simulink model "GFLIB_ControllerPIp_BAM"  (Simulink 9.3)
settings: Solver=VariableStepAuto  StartTime=0.0  StopTime=10.0  RelTol=1e-3
settings Model: Creator=nxa18952  LastModifiedBy=nxa18952
settings DataIOCC: SaveFormat=Dataset  SignalLoggingSaveFormat=Dataset  ReturnWorkspaceOutputs=on
settings OptimizationCC: LifeSpan=auto
settings DebuggingCC: UnderspecifiedInitializationDetection=Simplified  MergeDetectMultiDrivingBlocksExec=error  FcnCallInpInsideContextMsg=error  SFUnexpectedBacktrackingDiag=error  SFNoUnconditionalDefaultTransitionDiag=error  SFExecutionAtInitializationDiag=warning  ArithmeticOperatorsInVariantConditions=error
settings HardwareCC: ProdBitPerPointer=64  ProdBitPerSizeT=64  ProdBitPerPtrDiffT=64  ProdLargestAtomicFloat=Float  ProdIntDivRoundTo=Zero  ProdEndianess=LittleEndian  ProdWordSize=64  ProdHWDeviceType=Intel->x86-64 (Windows64)
settings ModelReferenceCC: PropagateSignalLabelsOutOfModel=on
settings SFSimCC: SimUseLocalCustomCode=on
settings RTWCC: RTWUseLocalCustomCode=on
settings CodeAppCC: StateflowObjectComments=off
settings GRTTargetCC: TargetLangStandard=C99 (ISO)  CombineOutputUpdateFcns=on  GRTInterface=off
settings ConfigComp: CovMetricSettings=dwe  CovHtmlReporting=off  CovSaveCumulativeToWorkspaceVar=off  CovSaveSingleToWorkspaceVar=off  CovExternalEMLEnable=on

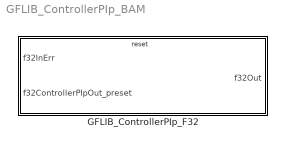
== system GFLIB_ControllerPIp_BAM ==
  GFLIB_ControllerPIp_F32 : Subsystem  TreatAsAtomicUnit=on  mask(GFLIB_ControllerPIp_F32){showStates=Hide (faster execution), resetStatesEnable=Pre-set according to the first set of inputs after reset, f32PropGain=0, f32IntegGain=0, s16PropGainShift=0, s16IntegGainShift=0}
      mask prompts: showStates "Show internal states"; resetStatesEnable "Internal state after reset"; f32PropGain "f32PropGain (Proportional gain)"; f32IntegGain "f32IntegGain (Integral gain)"; s16PropGainShift "s16PropGainShift (Proportional gain shift)"; s16IntegGainShift "s16IntegGainShift (Integral gain shift)"
      mask help: Parallel form PI controller without anti-windup in 32-bit fixed-point fractional implementation. This block supports re-initialization of the internal state during simulation. If the block is reset, the controller's output will be aligned with the input f32ControllerPIpOut_preset. Refer to the AMMCLIB User's Guide for further details.
      mask init:
      | if ~evalin('base','exist(''tS8'',''var'')')
      |   if (2 ~= exist('SWLIBS_Typedefs.mat','file'))
      |       error('File SWLIBS_Typedefs.mat is not on the Matlab path. Please add the AMMCLIB "bam" folder in the Matlab Search Path.');
      |   else
      |       evalin('base', 'load(''SWLIBS_Typedefs.mat'')');
      |   end
      | end
      | if showStates == 1
      |     % hidden state variables
      |     if strcmp(get_param([gcb '/f32PropGain'], 'BlockType'), 'Inport')
      |         posblk = get_param(gcb, 'Position');
      | 
      |         pos = get_param(    [gcb, '/f32PropGain'], 'Position');
      |         orient = get_param( [gcb, '/f32PropGain'], 'Orientation');
      |         delete_block(       [gcb, '/f32PropGain']);
      |         add_block('built-in/Ground', [gcb, '/f32PropGain'], 'Position', pos, 'Orientation', orient);
      | 
      |         pos = get_param(    [gcb, '/f32IntegGain'], 'Position');
      |         orient = get_param( [gcb, '/f32IntegGain'], 'Orientation');
      |         delete_block(       [gcb, '/f32IntegGain']);
      |         add_block('built-in/Ground', [gcb, '/f32IntegGain'], 'Position', pos, 'Orientation', orient);
      | 
      |         pos = get_param(    [gcb, '/s16PropGainShift'], 'Position');
      |         orient = get_param( [gcb, '/s16PropGainShift'], 'Orientation');
      |         delete_block(       [gcb, '/s16PropGainShift']);
      |         add_block('built-in/Ground', [gcb, '/s16PropGainShift'], 'Position', pos, 'Orientation', orient);
      | 
      |         pos = get_param(    [gcb, '/s16IntegGainShift'], 'Position');
      |         orient = get_param( [gcb, '/s16IntegGainShift'], 'Orientation');
      |         delete_block(       [gcb, '/s16IntegGainShift']);
      |         add_block('built-in/Ground', [gcb, '/s16IntegGainShift'], 'Position', pos, 'Orientation', orient);
      | 
      |         pos = get_param(    [gcb, '/f32IntegPartK_1'], 'Position');
      |         orient = get_param( [gcb, '/f32IntegPartK_1'], 'Orientation');
      |         delete_block(       [gcb, '/f32IntegPartK_1']);
      |         add_block('built-in/Ground', [gcb, '/f32IntegPartK_1'], 'Position', pos, 'Orientation', orient);
      | 
      |         pos = get_param(    [gcb, '/f32InK_1'], 'Position');
      |         orient = get_param( [gcb, '/f32InK_1'], 'Orientation');
      |         delete_block(       [gcb, '/f32InK_1']);
      |         add_block('built-in/Ground', [gcb, '/f32InK_1'], 'Position', pos, 'Orientation', orient);
      | 
      | 
      |         pos = get_param(    [gcb '/f32IntegPartK_1_Out'], 'Position');
      |         orient = get_param( [gcb '/f32IntegPartK_1_Out'], 'Orientation');
      |         delete_block(       [gcb '/f32IntegPartK_1_Out']);
      |         add_block('built-in/Terminator', [gcb '/f32IntegPartK_1_Out'], 'Position', pos, 'Orientation', orient);
      | 
      |         pos = get_param(    [gcb '/f32InK_1_Out'], 'Position');
      |         orient = get_param( [gcb '/f32InK_1_Out'], 'Orientation');
      |         delete_block(       [gcb '/f32InK_1_Out']);
      |         add_block('built-in/Terminator', [gcb '/f32InK_1_Out'], 'Position', pos, 'Orientation', orient);
      | 
      | 
      |         set_param([gcb '/f32InErr'], 'Port', '1');
      |         set_param([gcb '/f32ControllerPIpOut_preset'], 'Port', '2');
      | 
      |         set_param([gcb '/f32Out'], 'Port', '1');
      | 
      |         set_param(gcb,'MaskEnables',{'on','on','on','on','on','on'});
      | 
      |         if (posblk(4) - posblk(2)) > 75
      |           height = 75;
      |           set_param(gcb,'Position',[posblk(1), posblk(2), posblk(3), posblk(2)+height])
      |         end
      |     end
      | else
      |     % shown state variables
      |     if strcmp(get_param([gcb '/f32PropGain'], 'BlockType'), 'Ground')
      |         posblk = get_param(gcb, 'Position');
      | 
      |         pos = get_param(    [gcb, '/f32PropGain'], 'Position');
      |         orient = get_param( [gcb, '/f32PropGain'], 'Orientation');
      |         delete_block(       [gcb, '/f32PropGain']);
      |         add_block('built-in/Inport', [gcb, '/f32PropGain'], 'Position', pos, 'Orientation', orient, 'OutDataTypeStr', 'int32');
      | 
      |         pos = get_param(    [gcb, '/f32IntegGain'], 'Position');
      |         orient = get_param( [gcb, '/f32IntegGain'], 'Orientation');
      |         delete_block(       [gcb, '/f32IntegGain']);
      |         add_block('built-in/Inport', [gcb, '/f32IntegGain'], 'Position', pos, 'Orientation', orient, 'OutDataTypeStr', 'int32');
      | 
      |         pos = get_param(    [gcb, '/s16PropGainShift'], 'Position');
      |         orient = get_param( [gcb, '/s16PropGainShift'], 'Orientation');
      |         delete_block(       [gcb, '/s16PropGainShift']);
      |         add_block('built-in/Inport', [gcb, '/s16PropGainShift'], 'Position', pos, 'Orientation', orient, 'OutDataTypeStr', 'int16');
      | 
      |         pos = get_param(    [gcb, '/s16IntegGainShift'], 'Position');
      |         orient = get_param( [gcb, '/s16IntegGainShift'], 'Orientation');
      |         delete_block(       [gcb, '/s16IntegGainShift']);
      |         add_block('built-in/Inport', [gcb, '/s16IntegGainShift'], 'Position', pos, 'Orientation', orient, 'OutDataTypeStr', 'int16');
      | 
      |         pos = get_param(    [gcb, '/f32IntegPartK_1'], 'Position');
      |         orient = get_param( [gcb, '/f32IntegPartK_1'], 'Orientation');
      |         delete_block(       [gcb, '/f32IntegPartK_1']);
      |         add_block('built-in/Inport', [gcb, '/f32IntegPartK_1'], 'Position', pos, 'Orientation', orient, 'OutDataTypeStr', 'int32');
      | 
      |         pos = get_param(    [gcb, '/f32InK_1'], 'Position');
      |         orient = get_param( [gcb, '/f32InK_1'], 'Orientation');
      |         delete_block(       [gcb, '/f32InK_1']);
      |         add_block('built-in/Inport', [gcb, '/f32InK_1'], 'Position', pos, 'Orientation', orient, 'OutDataTypeStr', 'int32');
      | 
      | 
      |         pos = get_param(    [gcb '/f32IntegPartK_1_Out'], 'Position');
      |         orient = get_param( [gcb '/f32IntegPartK_1_Out'], 'Orientation');
      |         delete_block(       [gcb '/f32IntegPartK_1_Out']);
      |         add_block('built-in/Outport', [gcb '/f32IntegPartK_1_Out'], 'Position', pos, 'Orientation', orient);
      | 
      |         pos = get_param(    [gcb '/f32InK_1_Out'], 'Position');
      |         orient = get_param( [gcb '/f32InK_1_Out'], 'Orientation');
      |         delete_block(       [gcb '/f32InK_1_Out']);
      |         add_block('built-in/Outport', [gcb '/f32InK_1_Out'], 'Position', pos, 'Orientation', orient);
      | 
      | 
      |         set_param([gcb '/f32InErr'], 'Port', '1');
      |         set_param([gcb '/f32ControllerPIpOut_preset'], 'Port', '2');
      |         set_param([gcb '/f32PropGain'], 'Port', '3');
      |         set_param([gcb '/f32IntegGain'], 'Port', '4');
      |         set_param([gcb '/s16PropGainShift'], 'Port', '5');
      |         set_param([gcb '/s16IntegGainShift'], 'Port', '6');
      |         set_param([gcb '/f32IntegPartK_1'], 'Port', '7');
      |         set_param([gcb '/f32InK_1'], 'Port', '8');
      | 
      |         set_param([gcb '/f32Out'], 'Port', '1');
      |         set_param([gcb '/f32IntegPartK_1_Out'], 'Port', '2');
      |         set_param([gcb '/f32InK_1_Out'], 'Port', '3');
      | 
      |         set_param(gcb,'MaskEnables',{'on','on','off','off','off','off'});
      | 
      |         if (posblk(4) - posblk(2)) < 225
      |           height = 225;
      |           set_param(gcb,'Position',[posblk(1), posblk(2), posblk(3), posblk(2)+height])
      |         end
      |     end
      | end
      settings: RTWSystemCode=Inline
      mask TypeOptions showStates: Hide (faster execution) | Show (allows debugging; connect feedback loops manually)
      mask Callback showStates:
      | maskStr = get_param(gcb,'showStates');
      | if strcmp(maskStr,'Hide (faster execution)'),
      |     set_param(gcb,'MaskEnables',{'on','on','on','on','on','on'});
      | else
      |     set_param(gcb,'MaskEnables',{'on','on','off','off','off','off'});
      | end
      mask TypeOptions resetStatesEnable: Pre-set according to the first set of inputs after reset | Clear to zero
      mask Display:
      | color('black');
      | pos = get_param(gcb, 'Position');
      | width = pos(3) - pos(1);
      | height = pos(4) - pos(2);
      | tX=width/2;
      | tY=height - 25;
      | color('black');
      | text(tX,tY, 'GFLIB_ControllerPIp_F32', 'horizontalAlignment', 'center');
      | if showStates == 2
      |   color('red');
      |   text(tX,tY - 20, ['debugging mode' char(13) char(10) '(limited performance)'], 'horizontalAlignment', 'center');
      | end

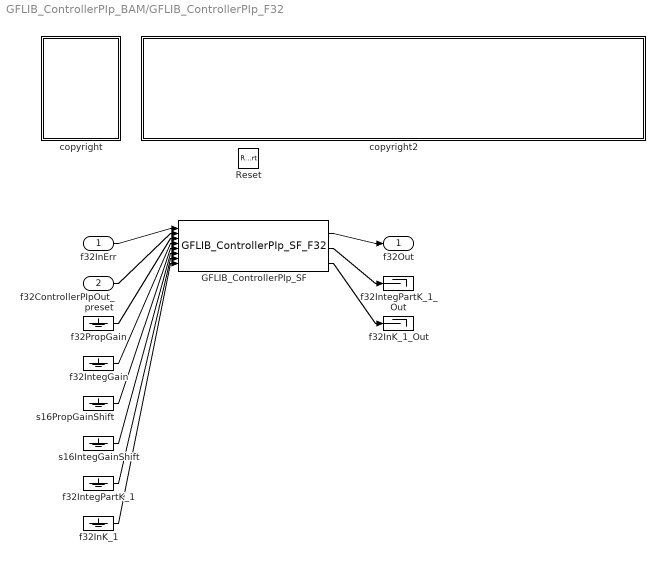
== system GFLIB_ControllerPIp_BAM/GFLIB_ControllerPIp_F32 ==
  f32InErr : Inport  OutDataTypeStr=int32
  f32ControllerPIpOut_preset : Inport  Port=2  OutDataTypeStr=int32
  Reset : ResetPort  DisableCoverage=on
  GFLIB_ControllerPIp_SF : S-Function  FunctionName=GFLIB_ControllerPIp_SF_F32  Parameters=showStates,resetStatesEnable,f32PropGain,f32IntegGain,s16PropGainShift,s16IntegGainShift  SFunctionDeploymentMode=off  EnableBusSupport=off
  copyright : Subsystem
      mask Display: text(10,90,'FILE:');text(10,75,'DESRIPTION:');text(10,60,'COPYRIGHT:');text(10,45,'VERSION:');text(10,30,'DATE:')
  copyright2 : Subsystem
      mask Display: text(10,90,'GFLIB_ControllerPIp_BAM_F32.mdl');text(10,75,'Parallel form of a standard PI controller without anti-windup.');text(10,60,'NXP 2020');text(10,45,'1.0');text(10,30,'28-Mar-2020');
  f32InK_1 : Ground
  f32InK_1_Out : Terminator
  f32IntegGain : Ground
  f32IntegPartK_1 : Ground
  f32IntegPartK_1_Out : Terminator
  f32PropGain : Ground
  s16IntegGainShift : Ground
  s16PropGainShift : Ground
  f32Out : Outport
  wires:
  f32InErr/1 -> GFLIB_ControllerPIp_SF/1
  f32ControllerPIpOut_preset/1 -> GFLIB_ControllerPIp_SF/2
  f32PropGain/1 -> GFLIB_ControllerPIp_SF/3
  f32IntegGain/1 -> GFLIB_ControllerPIp_SF/4
  s16PropGainShift/1 -> GFLIB_ControllerPIp_SF/5
  s16IntegGainShift/1 -> GFLIB_ControllerPIp_SF/6
  f32IntegPartK_1/1 -> GFLIB_ControllerPIp_SF/7
  f32InK_1/1 -> GFLIB_ControllerPIp_SF/8
  GFLIB_ControllerPIp_SF/1 -> f32Out/1
  GFLIB_ControllerPIp_SF/2 -> f32IntegPartK_1_Out/1
  GFLIB_ControllerPIp_SF/3 -> f32InK_1_Out/1

== system GFLIB_ControllerPIp_BAM/GFLIB_ControllerPIp_F32/copyright ==

== system GFLIB_ControllerPIp_BAM/GFLIB_ControllerPIp_F32/copyright2 ==
